simulink model "SCADA"  (R2021a)
settings: Solver=ode1  StartTime=0.0  StopTime=inf  FixedStep=0.001  RelTol=1e-3
InitFcn:
  | addpath('SCADA');
  | initFcn_SCADA;
model workspace (MAT data in the model file):
  RadSysCoeff = Simulink.Parameter
  RadSysCoeff.Value = [1 2 3 4]
  RadSysCoeff.DataType = 'auto'
  RadSysCoeff.Dimensions = [1 4]
values from neighbouring files (symbols this model uses):
  s = scatter(X(iVar),Y(iVar),100,[color(N-i+1,:)])    [postprocess_datafiles_accum_wRV.m]
undefined symbols (not defined in the file or in its folder): daq, g, HIL_act_A_cap, HIL_act_A_rod, HIL_charge_kd, HIL_charge_ki, HIL_charge_kp, HIL_charge_nMax, HIL_charge_nMin, HIL_ERU_kd, HIL_ERU_ki, HIL_ERU_kp, HIL_ERU_nMax, HIL_ERU_nMin, HIL_gen_kd, HIL_gen_ki, HIL_gen_kp, HIL_gen_nMax, HIL_gen_nMin, HIL_H1T_kp, HIL_H1T_negCutIn, HIL_H1T_posCutIn, HIL_scale_sys, HIL_WECpump_A_cap, HIL_WECpump_A_rod, HIL_WECpump_ang2lin, HIL_WECpump_negativeLimit, HIL_WECpump_positiveLimit, National_Instruments, PCIe, rho, wave_phi, wave_S_w, WEC_A_rad, WEC_B_rad, WEC_dw, WEC_F_amp, WEC_h, WEC_I, WEC_I_inf, WEC_ICs, WEC_L_cm, WEC_L_flap, WEC_m, WEC_phi_e, WEC_T, WEC_W, WEC_w
libraries: sldrtlib x21, daqlib x2, slpidlib x2, pid_lib x1, simulink x1
settings Model: Creator=Jeremy  LastModifiedBy=simmo536
settings RTWCC: BuildConfiguration=Faster Runs

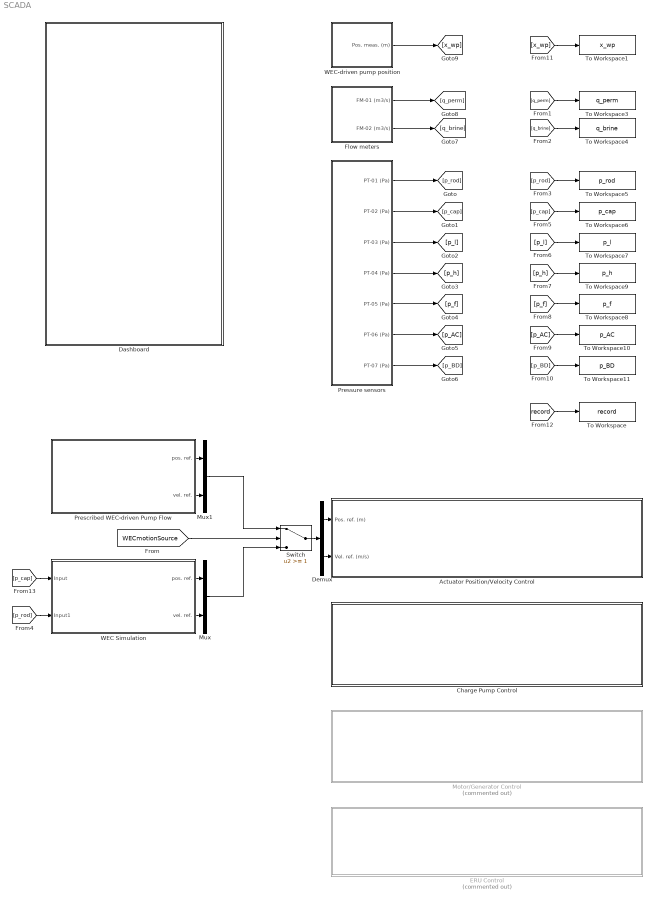
== system SCADA ==
  Actuator Position/Velocity Control : Subsystem
  Charge Pump Control : Subsystem
  Dashboard : Subsystem
  Demux : Demux  Outputs=2
  ERU Control : Subsystem  Commented=on
  Flow meters : Subsystem
  Motor/Generator Control : Subsystem  Commented=on
  Mux : Mux  Inputs=2
  Mux1 : Mux  Inputs=2
  Prescribed WEC-driven Pump Flow : Subsystem
  Pressure sensors : Subsystem
  Switch : Switch  Threshold=1
  To Workspace : ToWorkspace  VariableName=record  SaveFormat=Timeseries  SampleTime=-1
  To Workspace1 : ToWorkspace  VariableName=x_wp  SaveFormat=Timeseries  SampleTime=-1
  To Workspace10 : ToWorkspace  VariableName=p_AC  SaveFormat=Timeseries  SampleTime=-1
  To Workspace11 : ToWorkspace  VariableName=p_BD  SaveFormat=Timeseries  SampleTime=-1
  To Workspace3 : ToWorkspace  VariableName=q_perm  SaveFormat=Timeseries  SampleTime=-1
  To Workspace4 : ToWorkspace  VariableName=q_brine  SaveFormat=Timeseries  SampleTime=-1
  To Workspace5 : ToWorkspace  VariableName=p_rod  SaveFormat=Timeseries  SampleTime=-1
  To Workspace6 : ToWorkspace  VariableName=p_cap  SaveFormat=Timeseries  SampleTime=-1
  To Workspace7 : ToWorkspace  VariableName=p_l  SaveFormat=Timeseries  SampleTime=-1
  To Workspace8 : ToWorkspace  VariableName=p_f  SaveFormat=Timeseries  SampleTime=-1
  To Workspace9 : ToWorkspace  VariableName=p_h  SaveFormat=Timeseries  SampleTime=-1
  WEC Simulation : Subsystem
  WEC-driven pump position : Subsystem
  wires:
  WEC-driven pump position/1(Pos. meas. (m)) -> [x_wp]
  Pressure sensors/1(PT-01 (Pa)) -> [p_rod]
  Pressure sensors/2(PT-02 (Pa)) -> [p_cap]
  Pressure sensors/3(PT-03 (Pa)) -> [p_l]
  Pressure sensors/4(PT-04 (Pa)) -> [p_h]
  Pressure sensors/7(PT-07 (Pa)) -> [p_BD]
  Pressure sensors/6(PT-06 (Pa)) -> [p_AC]
  Pressure sensors/5(PT-05 (Pa)) -> [p_f]
  Flow meters/2(FM-02 (m3/s)) -> [q_brine]
  Flow meters/1(FM-01 (m3/s)) -> [q_perm]
  [record] -> To Workspace/1
  [x_wp] -> To Workspace1/1
  [q_perm] -> To Workspace3/1
  [p_rod] -> To Workspace5/1
  [q_brine] -> To Workspace4/1
  [p_cap] -> To Workspace6/1
  [p_l] -> To Workspace7/1
  [p_h] -> To Workspace9/1
  [p_f] -> To Workspace8/1
  [p_AC] -> To Workspace10/1
  [p_BD] -> To Workspace11/1
  [p_cap] -> WEC Simulation/1(Input)
  [p_rod] -> WEC Simulation/2(Input1)
  WEC Simulation/2(vel. ref.) -> Mux/2
  WEC Simulation/1(pos. ref.) -> Mux/1
  Demux/1 -> Actuator Position/Velocity Control/1(Pos. ref. (m))
  Demux/2 -> Actuator Position/Velocity Control/2(Vel. ref. (m/s))
  Switch/1 -> Demux/1
  [WECmotionSource] -> Switch/2
  Mux/1 -> Switch/3
  Prescribed WEC-driven Pump Flow/1(pos. ref.) -> Mux1/1
  Prescribed WEC-driven Pump Flow/2(vel. ref.) -> Mux1/2
  Mux1/1 -> Switch/1

== system SCADA/Actuator Position//Velocity Control ==
  Pos. ref. (m) : Inport
  Vel. ref. (m/s) : Inport  Port=2
  Derivative : Derivative
  Subsystem : Subsystem
  Transfer Fcn : TransferFcn  Denominator=[1/0.01 1]
  wires:
  [x_wp] -> Subsystem/3(Pos. meas. (m)), Derivative/1
  Derivative/1 -> Transfer Fcn/1
  Pos. ref. (m)/1 -> Subsystem/1(Pos. ref. (m))
  Vel. ref. (m/s)/1 -> Subsystem/2(Vel. ref. (m/s))
  Transfer Fcn/1 -> Subsystem/4(Vel. meas. (m/s))
  [H1T_shaftSpeed] -> Subsystem/5(H1T shaft speed (rpm))

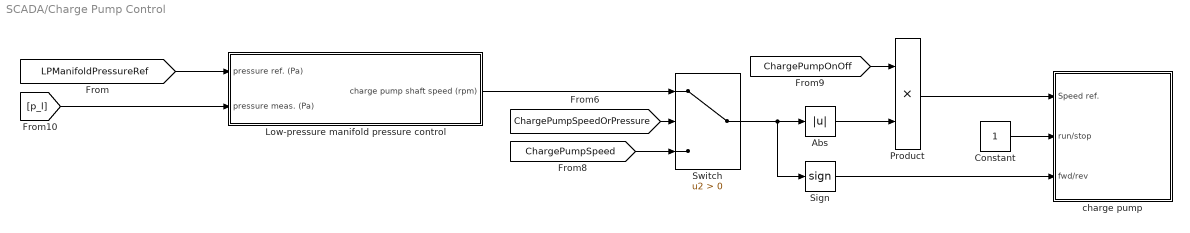
== system SCADA/Charge Pump Control ==
  Abs : Abs
  Constant : Constant
  Low-pressure manifold pressure control : Subsystem
  Product : Product
  Sign : Signum
  Switch : Switch  Criteria=u2 > Threshold
  charge pump : Subsystem
  wires:
  [p_l] -> Low-pressure manifold pressure control/2(pressure meas. (Pa))
  [ChargePumpSpeed] -> Switch/3
  Abs/1 -> Product/2
  Switch/1 -> Sign/1, Abs/1
  [LPManifoldPressureRef] -> Low-pressure manifold pressure control/1(pressure ref. (Pa))
  [ChargePumpOnOff] -> Product/1
  Low-pressure manifold pressure control/1(charge pump shaft speed (rpm)) -> Switch/1
  [ChargePumpSpeedOrPressure] -> Switch/2
  Product/1 -> charge pump/1(Speed ref.)
  Sign/1 -> charge pump/3(fwd/rev)
  Constant/1 -> charge pump/2(run/stop)

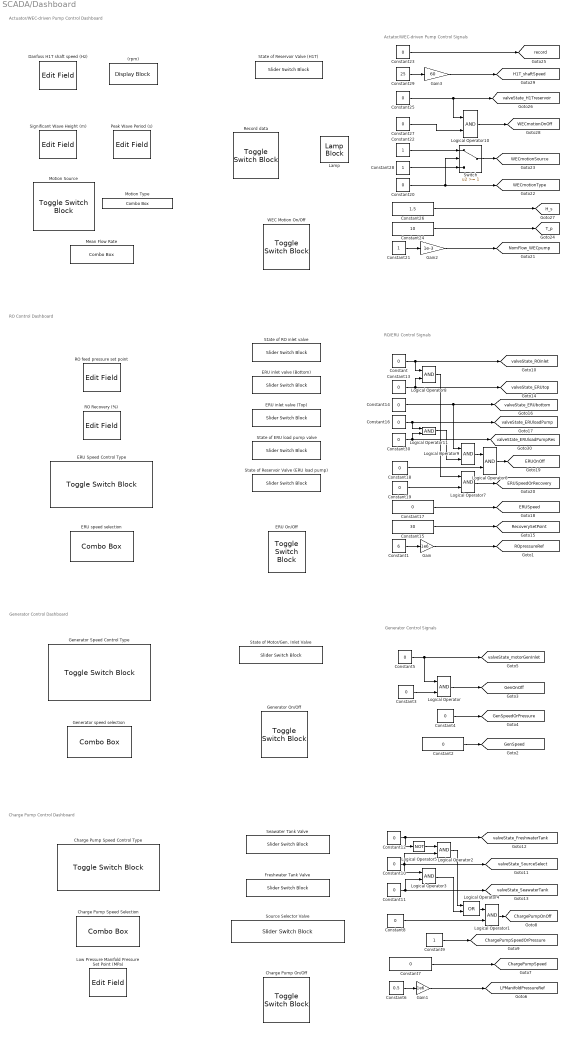
== system SCADA/Dashboard ==
  note: Charge Pump Control Dashboard
  note: Generator Control Signals
  note: RO Control Dashboard
  note: Generator Control Dashboard
  note: RO/ERU Control Signals
  note: Actuator/WEC-driven Pump Control Dashboard
  note: Actator/WEC-driven Pump Control Signals
  (rpm) : DisplayBlock  LabelPosition=Hide  Transparency=1
  Charge Pump On/Off : ToggleSwitchBlock  LabelPosition=Hide
      settings: Values={{'Off', 'On'}, [0 1]}
  Charge Pump Speed Control Type : ToggleSwitchBlock  LabelPosition=Hide
      settings: Values={{'Pressure control', 'Speed control'}, [1 0]}
  Charge Pump Speed Selection : ComboBox  LabelPosition=Hide  SelectedLabel=0 rpm
      settings: Values={{'0 rpm', '700 rpm', '1250 rpm', '2000 rpm', '2650 rpm', '3300 rpm'}, [0 700 1350 2000 2650 3300]}
  Constant{,2..5,7..8,10..14,16..20,23,25,27,30} (21 alike) : Constant  Value=0
  Constant1 : Constant  Value=6
  Constant15 : Constant  Value=30
  Constant{9,21..22,28} (4 alike) : Constant
  Constant24 : Constant  Value=10
  Constant26 : Constant  Value=1.5
  Constant29 : Constant  Value=25
  Constant6 : Constant  Value=0.5
  Danfoss H1T shaft speed (Hz) : EditField  LabelPosition=Hide  ShowInitialText=on  Alignment=Center
  ERU On/Off : ToggleSwitchBlock  LabelPosition=Hide
      settings: Values={{'Off', 'On'}, [0 1]}
  ERU Speed Control Type : ToggleSwitchBlock  LabelPosition=Hide
      settings: Values={{'Recovery control', 'Speed control'}, [1 0]}
  ERU inlet valve (Bottom) : SliderSwitchBlock  LabelPosition=Hide
      settings: Values={{'Closed', 'Open'}, [0 1]}
  ERU inlet valve (Top) : SliderSwitchBlock  LabelPosition=Hide
      settings: Values={{'Closed', 'Open'}, [0 1]}
  ERU speed selection : ComboBox  LabelPosition=Hide  SelectedLabel=0 rpm
      settings: Values={{'0 rpm', '500 rpm', '1000 rpm'}, [0 500 1000]}
  Freshwater Tank Valve : SliderSwitchBlock  LabelPosition=Hide
      settings: Values={{'Closed', 'Open'}, [0 1]}
  Gain : Gain  Gain=1e6
  Gain1 : Gain  Gain=1e6
  Gain2 : Gain  Gain=1e-3
  Gain3 : Gain  Gain=60
  Generator On/Off : ToggleSwitchBlock  LabelPosition=Hide
      settings: Values={{'Off', 'On'}, [0 1]}
  Generator Speed Control Type : ToggleSwitchBlock  LabelPosition=Hide
      settings: Values={{'Pressure control', 'Speed control'}, [1 0]}
  Generator speed selection : ComboBox  LabelPosition=Hide  SelectedLabel=0 rpm
      settings: Values={{'0 rpm', '500 rpm', '1000 rpm'}, [0 500 1000]}
  Lamp : LampBlock  LabelPosition=Hide
  Logical Operator{,1..3,6..11} (10 alike) : Logic  AllPortsSameDT=off  OutDataTypeStr=boolean
  Logical Operator4 : Logic  Operator=OR  AllPortsSameDT=off  OutDataTypeStr=boolean
  Logical Operator5 : Logic  Operator=NOT  AllPortsSameDT=off  OutDataTypeStr=boolean
  Low Pressure Manifold Pressure Set Point (MPa) : EditField  LabelPosition=Hide  ShowInitialText=on  Alignment=Center
  Mean Flow Rate : ComboBox  LabelPosition=Hide  SelectedLabel=1 L/s
      settings: Values={{'0 L/s', '1 L/s', '2 L/2'}, [0 1 2]}
  Motion Source : ToggleSwitchBlock  LabelPosition=Hide
      settings: Values={{'Prescribed', 'Simulation'}, [1 0]}
  Motion Type : ComboBox  LabelPosition=Hide  SelectedLabel=Constant Velocity
      settings: Values={{'Constant Velocity', 'Regular Waves', 'Irregular Waves'}, [0 1 2]}
  Peak Wave Period (s) : EditField  LabelPosition=Hide  ShowInitialText=on  Alignment=Center
  RO Recovery (%) : EditField  LabelPosition=Hide  ShowInitialText=on  Alignment=Center
  RO feed pressure set point : EditField  LabelPosition=Hide  ShowInitialText=on  Alignment=Center
  Record data : ToggleSwitchBlock  LabelPosition=Hide
      settings: Values={{'Off', 'On'}, [0 1]}
  Seawater Tank Valve : SliderSwitchBlock  LabelPosition=Hide
      settings: Values={{'Closed', 'Open'}, [0 1]}
  Significant Wave Height (m) : EditField  LabelPosition=Hide  ShowInitialText=on  Alignment=Center
  Source Selector Valve : SliderSwitchBlock  LabelPosition=Hide
      settings: Values={{'Freshwater', 'Seawater'}, [0 1]}
  State of ERU load pump valve : SliderSwitchBlock  LabelPosition=Hide
      settings: Values={{'Closed', 'Open'}, [0 1]}
  State of Motor/Gen. Inlet Valve : SliderSwitchBlock  LabelPosition=Hide
      settings: Values={{'Closed', 'Open'}, [0 1]}
  State of RO inlet valve : SliderSwitchBlock  LabelPosition=Hide
      settings: Values={{'Closed', 'Open'}, [0 1]}
  State of Reservoir Valve (ERU load pump) : SliderSwitchBlock  LabelPosition=Hide
      settings: Values={{'Closed', 'Open'}, [0 1]}
  State of Reservoir Valve (H1T) : SliderSwitchBlock  LabelPosition=Hide
      settings: Values={{'Closed', 'Open'}, [0 1]}
  Switch : Switch  Threshold=1
  WEC Motion On/Off : ToggleSwitchBlock  LabelPosition=Hide
      settings: Values={{'Off', 'On'}, [0 1]}
  tag scope: ChargePumpOnOff=global, ChargePumpSpeed=global, ChargePumpSpeedOrPressure=global, ERUOnOff=global, ERUSpeed=global, ERUSpeedOrRecovery=global, GenOnOff=global, GenSpeed=global, GenSpeedOrPressure=global, H1T_shaftSpeed=global, H_s=global, LPManifoldPressureRef=global, NomFlow_WECpump=global, ROpressureRef=global, RecoverySetPoint=global, T_p=global, WECmotionOnOff=global, WECmotionSource=global, WECmotionType=global, record=global, valveState_ERUbottom=global, valveState_ERUloadPump=global, valveState_ERUloadPumpRes=global, valveState_ERUtop=global, valveState_FreshwaterTank=global, valveState_H1Treservoir=global, valveState_ROinlet=global, valveState_SeawaterTank=global, valveState_SourceSelect=global, valveState_motorGenInlet=global
  wires:
  Constant/1 -> Logical Operator8/1, [valveState_ROinlet]
  Constant1/1 -> Gain/1
  Gain/1 -> [ROpressureRef]
  Constant2/1 -> [GenSpeed]
  Constant3/1 -> Logical Operator/2
  Constant4/1 -> [GenSpeedOrPressure]
  Constant5/1 -> Logical Operator/1, [valveState_motorGenInlet]
  Logical Operator/1 -> [GenOnOff]
  Logical Operator1/1 -> [ChargePumpOnOff]
  Constant9/1 -> [ChargePumpSpeedOrPressure]
  Constant10/1 -> [valveState_SourceSelect], Logical Operator2/2, Logical Operator3/1
  Gain1/1 -> [LPManifoldPressureRef]
  Constant6/1 -> Gain1/1
  Constant8/1 -> Logical Operator1/2
  Constant7/1 -> [ChargePumpSpeed]
  Constant12/1 -> Logical Operator5/1, [valveState_FreshwaterTank]
  Constant11/1 -> Logical Operator3/2, [valveState_SeawaterTank]
  Logical Operator4/1 -> Logical Operator1/1
  Logical Operator3/1 -> Logical Operator4/2
  Logical Operator2/1 -> Logical Operator4/1
  Logical Operator5/1 -> Logical Operator2/1
  Logical Operator6/1 -> [ERUOnOff]
  Constant17/1 -> [ERUSpeed]
  Constant13/1 -> Logical Operator8/2, [valveState_ERUtop]
  Constant19/1 -> Logical Operator7/2
  Constant18/1 -> Logical Operator6/2
  Constant14/1 -> [valveState_ERUbottom], Logical Operator9/1
  Constant15/1 -> [RecoverySetPoint]
  Logical Operator7/1 -> [ERUSpeedOrRecovery]
  Logical Operator8/1 -> Logical Operator7/1
  Logical Operator9/1 -> Logical Operator6/1
  Constant16/1 -> [valveState_ERUloadPump], Logical Operator11/1
  Constant24/1 -> [T_p]
  Constant26/1 -> [H_s]
  Logical Operator10/1 -> [WECmotionOnOff]
  Constant21/1 -> Gain2/1
  Constant25/1 -> Logical Operator10/1, [valveState_H1Treservoir]
  Gain2/1 -> [NomFlow_WECpump]
  Constant27/1 -> Logical Operator10/2
  Constant20/1 -> Switch/2, [WECmotionType]
  Constant22/1 -> Switch/1
  Constant23/1 -> [record]
  Constant28/1 -> Switch/3
  Switch/1 -> [WECmotionSource]
  Constant29/1 -> Gain3/1
  Gain3/1 -> [H1T_shaftSpeed]
  Constant30/1 -> [valveState_ERUloadPumpRes], Logical Operator11/2
  Logical Operator11/1 -> Logical Operator9/2

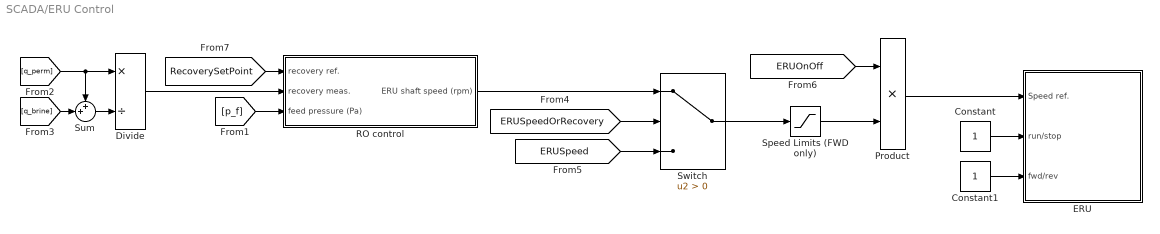
== system SCADA/ERU Control ==
  Constant : Constant
  Constant1 : Constant
  Divide : Product  Inputs=*/
  ERU : Subsystem
  Product : Product
  RO control : Subsystem
  Speed Limits (FWD only) : Saturate  UpperLimit=HIL_ERU_nMax  LowerLimit=HIL_ERU_nMin
  Sum : Sum  Inputs=++|
  Switch : Switch  Criteria=u2 > Threshold
  wires:
  Constant/1 -> ERU/2(run/stop)
  [p_f] -> RO control/3(feed pressure (Pa))
  [q_perm] -> Sum/1, Divide/1
  [q_brine] -> Sum/2
  Sum/1 -> Divide/2
  [RecoverySetPoint] -> RO control/1(recovery ref.)
  Divide/1 -> RO control/2(recovery meas.)
  [ERUSpeedOrRecovery] -> Switch/2
  Switch/1 -> Speed Limits (FWD only)/1
  [ERUSpeed] -> Switch/3
  RO control/1(ERU shaft speed (rpm)) -> Switch/1
  Speed Limits (FWD only)/1 -> Product/2
  [ERUOnOff] -> Product/1
  Product/1 -> ERU/1(Speed ref.)
  Constant1/1 -> ERU/3(fwd/rev)

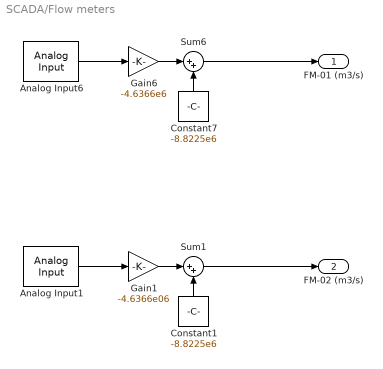
== system SCADA/Flow meters ==
  Analog Input1 : sldrtlib/Analog Input  SampleTime=0.1  MaxMissedTicks=10  ShowMissedTicks=off  YieldWhenWaiting=on  DrvName=National_Instruments/PCIe-6343  DrvAddress=4294967295  DrvOptions=[0 4367 12288 3 3 3 3]  Channels=7  RangeMode=1  VoltRange=1  DataType=1
      settings: AttributesFormatString=National Instruments\nPCIe-6343 [auto]
  Analog Input6 : sldrtlib/Analog Input  SampleTime=0.1  MaxMissedTicks=10  ShowMissedTicks=off  YieldWhenWaiting=on  DrvName=National_Instruments/PCIe-6343  DrvAddress=4294967295  DrvOptions=[0 4367 12288 3 3 3 3]  Channels=7  RangeMode=1  VoltRange=1  DataType=1
      settings: AttributesFormatString=National Instruments\nPCIe-6343 [auto]
  Constant1 : Constant  Value=-8.8225e6
  Constant7 : Constant  Value=-8.8225e6
  Gain1 : Gain  Gain=-4.6366e06
  Gain6 : Gain  Gain=-4.6366e6
  Sum1 : Sum  Inputs=|++
  Sum6 : Sum  Inputs=|++
  FM-01 (m3/s) : Outport
  FM-02 (m3/s) : Outport  Port=2
  wires:
  Constant7/1 -> Sum6/2
  Analog Input6/1 -> Gain6/1
  Gain6/1 -> Sum6/1
  Sum6/1 -> FM-01 (m3/s)/1
  Gain1/1 -> Sum1/1
  Sum1/1 -> FM-02 (m3/s)/1
  Constant1/1 -> Sum1/2
  Analog Input1/1 -> Gain1/1

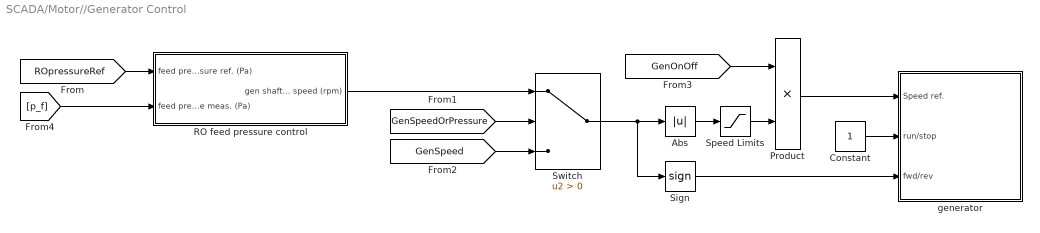
== system SCADA/Motor//Generator Control ==
  Abs : Abs
  Constant : Constant
  Product : Product
  RO feed pressure control : Subsystem
  Sign : Signum
  Speed Limits : Saturate  UpperLimit=HIL_gen_nMax  LowerLimit=HIL_gen_nMin
  Switch : Switch  Criteria=u2 > Threshold
  generator : Subsystem
  wires:
  RO feed pressure control/1(gen shaft speed (rpm)) -> Switch/1
  [p_f] -> RO feed pressure control/2(feed pressure meas. (Pa))
  [ROpressureRef] -> RO feed pressure control/1(feed pressure ref. (Pa))
  Switch/1 -> Sign/1, Abs/1
  [GenSpeedOrPressure] -> Switch/2
  [GenSpeed] -> Switch/3
  [GenOnOff] -> Product/1
  Product/1 -> generator/1(Speed ref.)
  Constant/1 -> generator/2(run/stop)
  Sign/1 -> generator/3(fwd/rev)
  Speed Limits/1 -> Product/2
  Abs/1 -> Speed Limits/1

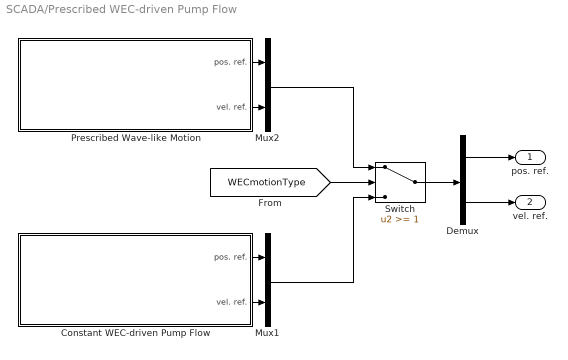
== system SCADA/Prescribed WEC-driven Pump Flow ==
  Constant WEC-driven Pump Flow : Subsystem
  Demux : Demux  Outputs=2
  Mux1 : Mux  Inputs=2
  Mux2 : Mux  Inputs=2
  Prescribed Wave-like Motion : Subsystem
  Switch : Switch  Threshold=1
  pos. ref. : Outport
  vel. ref. : Outport  Port=2
  wires:
  Prescribed Wave-like Motion/2(vel. ref.) -> Mux2/2
  Prescribed Wave-like Motion/1(pos. ref.) -> Mux2/1
  Mux2/1 -> Switch/1
  Demux/2 -> vel. ref./1
  Demux/1 -> pos. ref./1
  Constant WEC-driven Pump Flow/1(pos. ref.) -> Mux1/1
  Constant WEC-driven Pump Flow/2(vel. ref.) -> Mux1/2
  [WECmotionType] -> Switch/2
  Switch/1 -> Demux/1
  Mux1/1 -> Switch/3

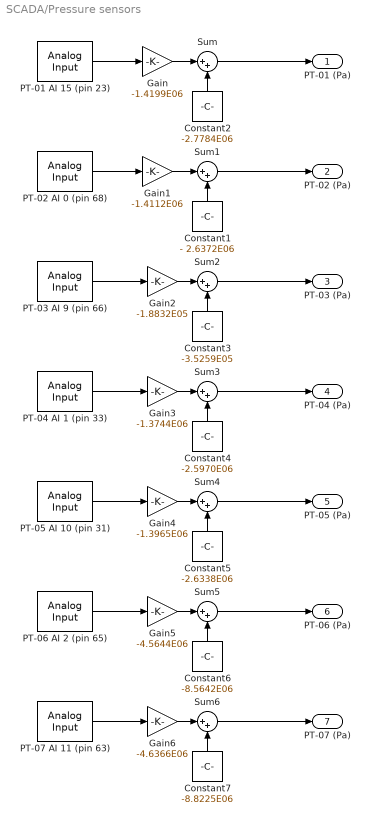
== system SCADA/Pressure sensors ==
  Constant1 : Constant  Value=- 2.6372E06
  Constant2 : Constant  Value=-2.7784E06
  Constant3 : Constant  Value=-3.5259E05
  Constant4 : Constant  Value=-2.5970E06
  Constant5 : Constant  Value=-2.6338E06
  Constant6 : Constant  Value=-8.5642E06
  Constant7 : Constant  Value=-8.8225E06
  Gain : Gain  Gain=-1.4199E06
  Gain1 : Gain  Gain=-1.4112E06
  Gain2 : Gain  Gain=-1.8832E05
  Gain3 : Gain  Gain=-1.3744E06
  Gain4 : Gain  Gain=-1.3965E06
  Gain5 : Gain  Gain=-4.5644E06
  Gain6 : Gain  Gain=-4.6366E06
  PT-01 AI 15 (pin 23) : sldrtlib/Analog Input  SampleTime=0.001  MaxMissedTicks=inf  ShowMissedTicks=off  YieldWhenWaiting=on  DrvName=National_Instruments/PCIe-6343  DrvAddress=4294967295  DrvOptions=[0 4367 12288 3 3 3 3]  Channels=16  RangeMode=1  VoltRange=1  DataType=1
      settings: AttributesFormatString=National Instruments\nPCIe-6343 [auto]
  PT-02 AI 0 (pin 68) : sldrtlib/Analog Input  SampleTime=0.1  MaxMissedTicks=inf  ShowMissedTicks=off  YieldWhenWaiting=on  DrvName=National_Instruments/PCIe-6343  DrvAddress=4294967295  DrvOptions=[0 4367 12288 3 3 3 3]  Channels=1  RangeMode=1  VoltRange=1  DataType=1
      settings: AttributesFormatString=National Instruments\nPCIe-6343 [auto]
  PT-03 AI 9 (pin 66) : sldrtlib/Analog Input  SampleTime=0.1  MaxMissedTicks=inf  ShowMissedTicks=off  YieldWhenWaiting=on  DrvName=National_Instruments/PCIe-6343  DrvAddress=4294967295  DrvOptions=[0 4367 12288 3 3 3 3]  Channels=10  RangeMode=1  VoltRange=1  DataType=1
      settings: AttributesFormatString=National Instruments\nPCIe-6343 [auto]
  PT-04 AI 1 (pin 33) : sldrtlib/Analog Input  SampleTime=0.1  MaxMissedTicks=10  ShowMissedTicks=off  YieldWhenWaiting=on  DrvName=National_Instruments/PCIe-6343  DrvAddress=4294967295  DrvOptions=[0 4367 12288 3 3 3 3]  Channels=2  RangeMode=1  VoltRange=1  DataType=1
      settings: AttributesFormatString=National Instruments\nPCIe-6343 [auto]
  PT-05 AI 10 (pin 31) : sldrtlib/Analog Input  SampleTime=0.1  MaxMissedTicks=inf  ShowMissedTicks=off  YieldWhenWaiting=on  DrvName=National_Instruments/PCIe-6343  DrvAddress=4294967295  DrvOptions=[0 4367 12288 3 3 3 3]  Channels=11  RangeMode=1  VoltRange=1  DataType=1
      settings: AttributesFormatString=National Instruments\nPCIe-6343 [auto]
  PT-06 AI 2 (pin 65) : sldrtlib/Analog Input  SampleTime=0.1  MaxMissedTicks=10  ShowMissedTicks=off  YieldWhenWaiting=on  DrvName=National_Instruments/PCIe-6343  DrvAddress=4294967295  DrvOptions=[0 4367 12288 3 3 3 3]  Channels=3  RangeMode=1  VoltRange=1  DataType=1
      settings: AttributesFormatString=National Instruments\nPCIe-6343 [auto]
  PT-07 AI 11 (pin 63) : sldrtlib/Analog Input  SampleTime=0.1  MaxMissedTicks=10  ShowMissedTicks=off  YieldWhenWaiting=on  DrvName=National_Instruments/PCIe-6343  DrvAddress=4294967295  DrvOptions=[0 4367 12288 3 3 3 3]  Channels=12  RangeMode=1  VoltRange=1  DataType=1
      settings: AttributesFormatString=National Instruments\nPCIe-6343 [auto]
  Sum{,1..6} (7 alike) : Sum  Inputs=|++
  PT-01 (Pa) : Outport
  PT-02 (Pa) : Outport  Port=2
  PT-03 (Pa) : Outport  Port=3
  PT-04 (Pa) : Outport  Port=4
  PT-05 (Pa) : Outport  Port=5
  PT-06 (Pa) : Outport  Port=6
  PT-07 (Pa) : Outport  Port=7
  wires:
  PT-01 AI 15 (pin 23)/1 -> Gain/1
  Constant2/1 -> Sum/2
  Sum/1 -> PT-01 (Pa)/1
  Sum1/1 -> PT-02 (Pa)/1
  Sum2/1 -> PT-03 (Pa)/1
  Sum3/1 -> PT-04 (Pa)/1
  Sum4/1 -> PT-05 (Pa)/1
  Sum5/1 -> PT-06 (Pa)/1
  Gain/1 -> Sum/1
  PT-02 AI 0 (pin 68)/1 -> Gain1/1
  Constant1/1 -> Sum1/2
  Gain1/1 -> Sum1/1
  PT-03 AI 9 (pin 66)/1 -> Gain2/1
  Constant3/1 -> Sum2/2
  Gain2/1 -> Sum2/1
  PT-04 AI 1 (pin 33)/1 -> Gain3/1
  Constant4/1 -> Sum3/2
  Gain3/1 -> Sum3/1
  PT-05 AI 10 (pin 31)/1 -> Gain4/1
  Constant5/1 -> Sum4/2
  Gain4/1 -> Sum4/1
  PT-06 AI 2 (pin 65)/1 -> Gain5/1
  Constant6/1 -> Sum5/2
  Gain5/1 -> Sum5/1
  PT-07 AI 11 (pin 63)/1 -> Gain6/1
  Sum6/1 -> PT-07 (Pa)/1
  Constant7/1 -> Sum6/2
  Gain6/1 -> Sum6/1

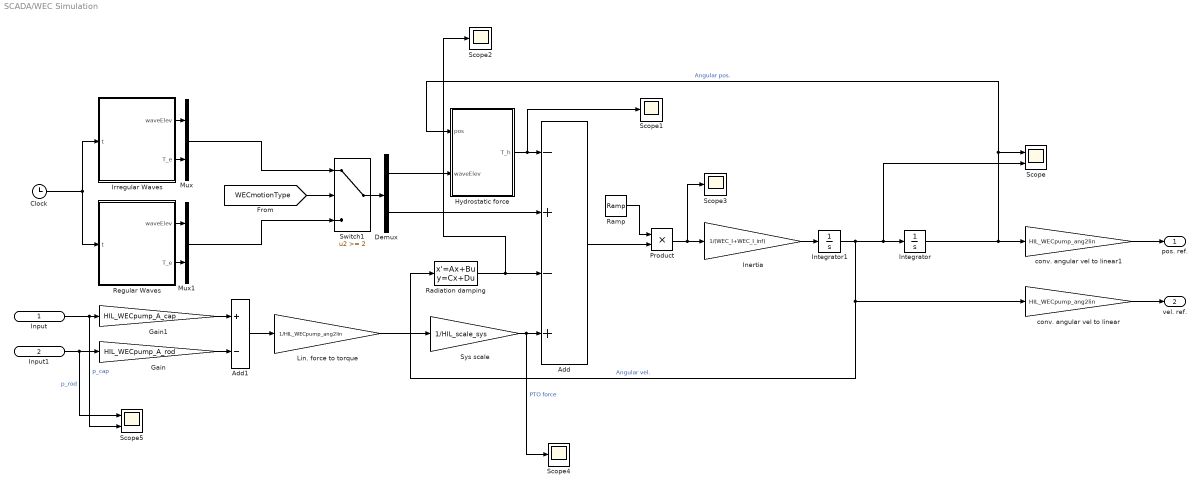
== system SCADA/WEC Simulation ==
  Input : Inport
  Input1 : Inport  Port=2
  Add : Sum  Inputs=-+-+
  Add1 : Sum  Inputs=+-
  Clock : Clock
  Demux : Demux  Outputs=2
  Gain : Gain  Gain=HIL_WECpump_A_rod
  Gain1 : Gain  Gain=HIL_WECpump_A_cap
  Hydrostatic force : MATLAB Function  TreatAsAtomicUnit=on
  Inertia : Gain  Gain=1/(WEC_I+WEC_I_inf)
  Integrator : Integrator
  Integrator1 : Integrator
  Irregular Waves : MATLAB Function  TreatAsAtomicUnit=on
  Lin. force to torque : Gain  Gain=1/HIL_WECpump_ang2lin
  Mux : Mux  Inputs=2
  Mux1 : Mux  Inputs=2
  Product : Product
  Radiation damping : StateSpace  A=WEC_A_rad  B=WEC_B_rad  C=[1,0,0]  D=0  InitialCondition=WEC_ICs
  Ramp : simulink/Sources/Ramp  slope=1/5  start=5  InitialOutput=0
  Regular Waves : MATLAB Function  TreatAsAtomicUnit=on
  Scope : Scope  NumInputPorts=2
  Scope{1..4} (4 alike) : Scope
  Scope5 : Scope  NumInputPorts=2
  Switch1 : Switch  Threshold=2
  Sys scale : Gain  Gain=1/HIL_scale_sys
  conv. angular vel to linear : Gain  Gain=HIL_WECpump_ang2lin
  conv. angular vel to linear1 : Gain  Gain=HIL_WECpump_ang2lin
  pos. ref. : Outport
  vel. ref. : Outport  Port=2
  wires:
  Radiation damping/1 -> Scope2/1, Add/3
  Clock/1 -> Regular Waves/1(t), Irregular Waves/1(t)
  Irregular Waves/1(waveElev) -> Mux/1
  Irregular Waves/2(T_e) -> Mux/2
  Hydrostatic force/1(T_h) -> Scope1/1, Add/1
  Inertia/1 -> Integrator1/1
  Integrator1/1 -> Scope/2, Integrator/1, Radiation damping/1, conv. angular vel to linear/1  "Angular vel."
  Integrator/1 -> conv. angular vel to linear1/1, Scope/1, Hydrostatic force/1(pos)  "Angular pos."
  Lin. force to torque/1 -> Sys scale/1
  Add1/1 -> Lin. force to torque/1
  Input/1 -> Scope5/2, Gain1/1  "p_cap"
  Input1/1 -> Scope5/1, Gain/1  "p_rod"
  conv. angular vel to linear1/1 -> pos. ref./1
  conv. angular vel to linear/1 -> vel. ref./1
  Sys scale/1 -> Scope4/1, Add/4  "PTO force"
  Gain/1 -> Add1/2
  Gain1/1 -> Add1/1
  Demux/1 -> Hydrostatic force/2(waveElev)
  [WECmotionType] -> Switch1/2
  Demux/2 -> Add/2
  Regular Waves/1(waveElev) -> Mux1/1
  Regular Waves/2(T_e) -> Mux1/2
  Switch1/1 -> Demux/1
  Mux1/1 -> Switch1/3
  Mux/1 -> Switch1/1
  Product/1 -> Scope3/1, Inertia/1
  Add/1 -> Product/2
  Ramp/1 -> Product/1

== system SCADA/WEC-driven pump position ==
  Analog Input : sldrtlib/Analog Input  SampleTime=0.1  MaxMissedTicks=inf  ShowMissedTicks=off  YieldWhenWaiting=on  DrvName=National_Instruments/PCIe-6343  DrvAddress=4294967295  DrvOptions=[0 4367 12288 3 3 3 3]  Channels=7  RangeMode=1  VoltRange=1  DataType=1
      settings: AttributesFormatString=National Instruments\nPCIe-6343 [auto]
  Constant2 : Constant  Value=2.5
  Gain : Gain  Gain=.1013
  Scope : Scope
  Sum : Sum  Inputs=|+-
  Pos. meas. (m) : Outport
  wires:
  Constant2/1 -> Sum/2
  Sum/1 -> Gain/1
  Gain/1 -> Pos. meas. (m)/1  "Pos (m)"
  Analog Input/1 -> Scope/1, Sum/1

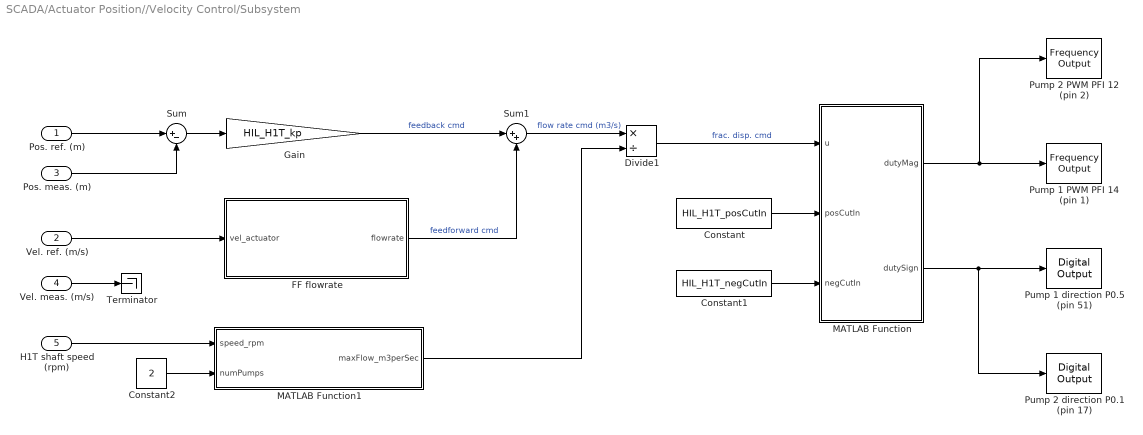
== system SCADA/Actuator Position//Velocity Control/Subsystem ==
  Pos. ref. (m) : Inport
  Vel. ref. (m/s) : Inport  Port=2
  Pos. meas. (m) : Inport  Port=3
  Vel. meas. (m/s) : Inport  Port=4
  H1T shaft speed (rpm) : Inport  Port=5
  Constant : Constant  Value=HIL_H1T_posCutIn
  Constant1 : Constant  Value=HIL_H1T_negCutIn
  Constant2 : Constant  Value=2
  Divide1 : Product  Inputs=*/
  FF flowrate : MATLAB Function  TreatAsAtomicUnit=on
  Gain : Gain  Gain=HIL_H1T_kp
  MATLAB Function : MATLAB Function  TreatAsAtomicUnit=on
  MATLAB Function1 : MATLAB Function  TreatAsAtomicUnit=on
  Pump 1 PWM PFI 14 (pin 1) : sldrtlib/Frequency Output  SampleTime=0.1  MaxMissedTicks=inf  ShowMissedTicks=off  YieldWhenWaiting=off  DrvName=National_Instruments/PCIe-6343  DrvAddress=4294967295  DrvOptions=[0 4367 12288 3 3 3 3]  Channels=3  FrequencySource=1  Frequency=100  FrequencyFinalValue=[]  DutySource=2  Duty=0  DutyFinalValue=0
      settings: AttributesFormatString=National Instruments\nPCIe-6343 [auto]  SourceProductBaseCode=WT
  Pump 1 direction P0.5 (pin 51) : sldrtlib/Digital Output  SampleTime=0.1  MaxMissedTicks=10  ShowMissedTicks=off  YieldWhenWaiting=off  DrvName=National_Instruments/PCIe-6343  DrvAddress=4294967295  DrvOptions=[0 4367 12288 3 3 3 3]  Channels=6  BitMode=1  InitialValue=1  FinalValue=1
      settings: AttributesFormatString=National Instruments\nPCIe-6343 [auto]  SourceProductBaseCode=WT
  Pump 2 PWM PFI 12 (pin 2) : sldrtlib/Frequency Output  SampleTime=0.1  MaxMissedTicks=inf  ShowMissedTicks=off  YieldWhenWaiting=off  DrvName=National_Instruments/PCIe-6343  DrvAddress=4294967295  DrvOptions=[0 4367 12288 3 3 3 3]  Channels=2  FrequencySource=1  Frequency=100  FrequencyFinalValue=[]  DutySource=2  Duty=0  DutyFinalValue=0
      settings: AttributesFormatString=National Instruments\nPCIe-6343 [auto]  SourceProductBaseCode=WT
  Pump 2 direction P0.1 (pin 17) : sldrtlib/Digital Output  SampleTime=0.1  MaxMissedTicks=10  ShowMissedTicks=off  YieldWhenWaiting=off  DrvName=National_Instruments/PCIe-6343  DrvAddress=4294967295  DrvOptions=[0 4367 12288 3 3 3 3]  Channels=1  BitMode=1  InitialValue=0  FinalValue=0
      settings: AttributesFormatString=National Instruments\nPCIe-6343 [auto]  SourceProductBaseCode=WT
  Sum : Sum  Inputs=|+-
  Sum1 : Sum  Inputs=|++
  Terminator : Terminator
  wires:
  FF flowrate/1(flowrate) -> Sum1/2  "feedforward cmd"
  Pos. meas. (m)/1 -> Sum/2
  MATLAB Function1/1(maxFlow_m3perSec) -> Divide1/2
  Constant2/1 -> MATLAB Function1/2(numPumps)
  Divide1/1 -> MATLAB Function/1(u)  "frac. disp. cmd"
  H1T shaft speed (rpm)/1 -> MATLAB Function1/1(speed_rpm)
  MATLAB Function/1(dutyMag) -> Pump 1 PWM PFI 14 (pin 1)/1, Pump 2 PWM PFI 12 (pin 2)/1
  Constant1/1 -> MATLAB Function/3(negCutIn)
  Sum1/1 -> Divide1/1  "flow rate cmd (m3/s)"
  Pos. ref. (m)/1 -> Sum/1
  Vel. ref. (m/s)/1 -> FF flowrate/1(vel_actuator)
  Gain/1 -> Sum1/1  "feedback cmd"
  MATLAB Function/2(dutySign) -> Pump 2 direction P0.1 (pin 17)/1, Pump 1 direction P0.5 (pin 51)/1
  Vel. meas. (m/s)/1 -> Terminator/1
  Sum/1 -> Gain/1
  Constant/1 -> MATLAB Function/2(posCutIn)

== system SCADA/Charge Pump Control/Low-pressure manifold pressure control ==
  pressure ref. (Pa) : Inport
  pressure meas. (Pa) : Inport  Port=2
  PID Controller : pid_lib/PID Controller  Controller=PI  Form=Parallel  TimeDomain=Continuous-time  UseExternalTs=off  SampleTime=-1  IntegratorMethod=Forward Euler  FilterMethod=Forward Euler  ControllerParametersSource=internal  P=HIL_charge_kp  I=HIL_charge_ki  D=HIL_charge_kd  UseFilter=on  N=100  TunerSelectOption=Transfer Function Based (PID Tuner App)  InitialConditionSource=internal  InitialConditionForIntegrator=0  InitialConditionForFilter=0  DifferentiatorICPrevScaledInput=0  ExternalReset=none  TrackingMode=off  Kt=1  LimitOutput=off  SatLimitsSource=internal  UpperSaturationLimit=inf  LowerSaturationLimit=-inf  LinearizeAsGain=on  AntiWindupMode=none  Kb=1  POutMin=[]  POutMax=[]  IOutMin=[]  IOutMax=[]  DOutMin=[]  DOutMax=[]  NOutMin=[]  NOutMax=[]  SumOutMin=[]  SumOutMax=[]  SaturationOutMin=[]  SaturationOutMax=[]  PParamMin=[]  PParamMax=[]  IParamMin=[]  IParamMax=[]  DParamMin=[]  DParamMax=[]  NParamMin=[]  NParamMax=[]  KbParamMin=[]  KbParamMax=[]  KtParamMin=[]  KtParamMax=[]  KbOutMin=[]  KbOutMax=[]  KtOutMin=[]  KtOutMax=[]  IntegratorOutMin=[]  IntegratorOutMax=[]  FilterOutMin=[]  FilterOutMax=[]  SumI1OutMin=[]  SumI1OutMax=[]  SumI2OutMin=[]  SumI2OutMax=[]  SumI3OutMin=[]  SumI3OutMax=[]  SumI4OutMin=[]  SumI4OutMax=[]  SumDOutMin=[]  SumDOutMax=[]  DifferentiatorOutMin=[]  DifferentiatorOutMax=[]  FilterDiffOutCoefMin=[]  FilterDiffOutCoefMax=[]  ReciprocalOutMin=[]  ReciprocalOutMax=[]  SumDenOutMin=[]  SumDenOutMax=[]  SumNumOutMin=[]  SumNumOutMax=[]  DivideOutMin=[]  DivideOutMax=[]  UdiffTsProdOutMin=[]  UdiffTsProdOutMax=[]  NTsProdOutMin=[]  NTsProdOutMax=[]  UintegralTsProdOutMin=[]  UintegralTsProdOutMax=[]  UngainTsProdOutMin=[]  UngainTsProdOutMax=[]  IntegratorContinuousStateAttributes=''  IntegratorStateMustResolveToSignalObject=off  IntegratorRTWStateStorageClass=Auto  FilterContinuousStateAttributes=''  FilterStateMustResolveToSignalObject=off  FilterRTWStateStorageClass=Auto  ParallelPVariant=InternalParameters  IdealPVariant=Disabled  IVariant=InternalParameters  DVariant=Disabled  IntegratorVariant=Continuous  SatVariant=Disabled  AWVariant=Passthrough  PCopyVariant=Disabled  TRVariant=Disabled  FdbkBlocksVariant=Forward  IdealPFdbkVariant=Disabled  SatFdbkVariant=Disabled  DerivativeFilterVariant=Disabled  NVariant=Disabled  NCopyVariant=Disabled_SignalSpec  FilterICVariant=Disabled  IntegratorICVariant=InternalICs  ExternalResetVariant=Disabled  TRSumVariant=Passthrough  SumFdbkVariant=Disabled  SumVariant=Sum_PI  TsampFilterVariant=InternalTs  TsampNgainVariant=Passthrough  TsampIntegralVariant=Passthrough  ExternalSaturationOutDataTypeStr=Inherit: Same as second input
  Speed Limits (FWD only) : Saturate  UpperLimit=HIL_charge_nMax  LowerLimit=HIL_charge_nMin
  Sum : Sum  Inputs=|+-
  charge pump shaft speed (rpm) : Outport
  wires:
  Sum/1 -> PID Controller/1
  PID Controller/1 -> Speed Limits (FWD only)/1  "feedback cmd"
  pressure ref. (Pa)/1 -> Sum/1
  pressure meas. (Pa)/1 -> Sum/2
  Speed Limits (FWD only)/1 -> charge pump shaft speed (rpm)/1

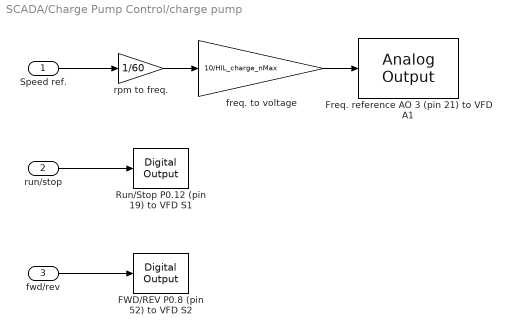
== system SCADA/Charge Pump Control/charge pump ==
  Speed ref. : Inport
  run/stop : Inport  Port=2
  fwd/rev : Inport  Port=3
  FWD/REV P0.8 (pin 52) to VFD S2 : sldrtlib/Digital Output  SampleTime=0.1  MaxMissedTicks=10  ShowMissedTicks=off  YieldWhenWaiting=off  DrvName=National_Instruments/PCIe-6343  DrvAddress=4294967295  DrvOptions=[0 4367 12288 3 3 3 3]  Channels=9  BitMode=1  InitialValue=0  FinalValue=0
      settings: AttributesFormatString=National Instruments\nPCIe-6343 [auto]  SourceProductBaseCode=WT
  "Freq. reference AO 3 (pin 21) to VFD A1 " : sldrtlib/Analog Output  SampleTime=0.1  MaxMissedTicks=inf  ShowMissedTicks=off  YieldWhenWaiting=off  DrvName=National_Instruments/PCIe-6343  DrvAddress=4294967295  DrvOptions=[0 4367 12288 3 3 3 3]  Channels=4  RangeMode=1  VoltRange=1  InitialValue=0  FinalValue=0
      settings: AttributesFormatString=National Instruments\nPCIe-6343 [auto]
  Run/Stop P0.12 (pin 19) to VFD S1 : sldrtlib/Digital Output  SampleTime=0.1  MaxMissedTicks=10  ShowMissedTicks=off  YieldWhenWaiting=off  DrvName=National_Instruments/PCIe-6343  DrvAddress=4294967295  DrvOptions=[0 4367 12288 3 3 3 3]  Channels=1  BitMode=1  InitialValue=[]  FinalValue=[]
      settings: AttributesFormatString=National Instruments\nPCIe-6343 [auto]  SourceProductBaseCode=WT
  freq. to voltage : Gain  Gain=10/HIL_charge_nMax
  rpm to freq. : Gain  Gain=1/60
  wires:
  Speed ref./1 -> rpm to freq./1
  rpm to freq./1 -> freq. to voltage/1
  freq. to voltage/1 -> "Freq. reference AO 3 (pin 21) to VFD A1 "/1
  run/stop/1 -> Run/Stop P0.12 (pin 19) to VFD S1/1
  fwd/rev/1 -> FWD/REV P0.8 (pin 52) to VFD S2/1

== system SCADA/ERU Control/ERU ==
  Speed ref. : Inport
  run/stop : Inport  Port=2
  fwd/rev : Inport  Port=3
  FWD/REV PFI 11/P2.3 (pin 46) to VFD S2 : sldrtlib/Digital Output  SampleTime=0.1  MaxMissedTicks=10  ShowMissedTicks=off  YieldWhenWaiting=off  DrvAddress=0  DrvOptions=0  Channels=1  BitMode=1  InitialValue=[]  FinalValue=[]
      settings: SourceProductBaseCode=WT
  "Freq. reference AO 0 (pin 22) to VFD A1 " : daqlib/Analog Output  DeviceMenu=(none)  Device=(none)  NChannelsSelected=1  NPorts=1 for all channels  SampleRate=0  ActualRate=0
      settings: SourceProductBaseCode=DA
  Run/Stop P0.3 (pin 47) to VFD S1 : sldrtlib/Digital Output  SampleTime=0.1  MaxMissedTicks=10  ShowMissedTicks=off  YieldWhenWaiting=off  DrvAddress=0  DrvOptions=0  Channels=1  BitMode=1  InitialValue=[]  FinalValue=[]
      settings: SourceProductBaseCode=WT
  freq. to voltage1 : Gain  Gain=10/HIL_ERU_nMax
  rpm to freq.1 : Gain  Gain=1/60
  wires:
  freq. to voltage1/1 -> "Freq. reference AO 0 (pin 22) to VFD A1 "/1
  run/stop/1 -> Run/Stop P0.3 (pin 47) to VFD S1/1
  fwd/rev/1 -> FWD/REV PFI 11/P2.3 (pin 46) to VFD S2/1
  rpm to freq.1/1 -> freq. to voltage1/1
  Speed ref./1 -> rpm to freq.1/1

== system SCADA/ERU Control/RO control ==
  recovery ref. : Inport
  recovery meas. : Inport  Port=2
  feed pressure (Pa) : Inport  Port=3
  PID Controller : slpidlib/PID Controller  Controller=PID  Form=Parallel  TimeDomain=Continuous-time  UseExternalTs=off  SampleTime=-1  IntegratorMethod=Forward Euler  FilterMethod=Forward Euler  ControllerParametersSource=internal  P=HIL_ERU_kp  I=HIL_ERU_ki  UseKiTs=off  D=HIL_ERU_kd  N=100  UseFilter=on  TunerSelectOption=Transfer Function Based (PID Tuner App)  InitialConditionSource=internal  InitialConditionForIntegrator=0  InitialConditionForFilter=0  DifferentiatorICPrevScaledInput=0  ExternalReset=none  TrackingMode=off  Kt=1  LimitOutput=off  SatLimitsSource=internal  UpperSaturationLimit=inf  LowerSaturationLimit=-inf  LinearizeAsGain=on  AntiWindupMode=none  Kb=1  POutMin=[]  POutMax=[]  IOutMin=[]  IOutMax=[]  DOutMin=[]  DOutMax=[]  NOutMin=[]  NOutMax=[]  SumOutMin=[]  SumOutMax=[]  SaturationOutMin=[]  SaturationOutMax=[]  PParamMin=[]  PParamMax=[]  IParamMin=[]  IParamMax=[]  DParamMin=[]  DParamMax=[]  NParamMin=[]  NParamMax=[]  KbParamMin=[]  KbParamMax=[]  KtParamMin=[]  KtParamMax=[]  KbOutMin=[]  KbOutMax=[]  KtOutMin=[]  KtOutMax=[]  IntegratorOutMin=[]  IntegratorOutMax=[]  FilterOutMin=[]  FilterOutMax=[]  SumI1OutMin=[]  SumI1OutMax=[]  SumI2OutMin=[]  SumI2OutMax=[]  SumI3OutMin=[]  SumI3OutMax=[]  SumI4OutMin=[]  SumI4OutMax=[]  SumDOutMin=[]  SumDOutMax=[]  DifferentiatorOutMin=[]  DifferentiatorOutMax=[]  FilterDiffOutCoefMin=[]  FilterDiffOutCoefMax=[]  ReciprocalOutMin=[]  ReciprocalOutMax=[]  SumDenOutMin=[]  SumDenOutMax=[]  SumNumOutMin=[]  SumNumOutMax=[]  DivideOutMin=[]  DivideOutMax=[]  UdiffTsProdOutMin=[]  UdiffTsProdOutMax=[]  NTsProdOutMin=[]  NTsProdOutMax=[]  UintegralTsProdOutMin=[]  UintegralTsProdOutMax=[]  UngainTsProdOutMin=[]  UngainTsProdOutMax=[]  IntegratorContinuousStateAttributes=''  IntegratorStateMustResolveToSignalObject=off  IntegratorRTWStateStorageClass=Auto  FilterContinuousStateAttributes=''  FilterStateMustResolveToSignalObject=off  FilterRTWStateStorageClass=Auto  ParallelPVariant=InternalParameters  IdealPVariant=Disabled  IVariant=InternalParameters  DVariant=InternalParameters  IntegratorVariant=Continuous  SatVariant=Disabled  AWVariant=Passthrough  PCopyVariant=Disabled  TRVariant=Disabled  FdbkBlocksVariant=Forward  IdealPFdbkVariant=Disabled  SatFdbkVariant=Disabled  DerivativeFilterVariant=ContFilter  NVariant=InternalParameters  NCopyVariant=Disabled  FilterICVariant=InternalICsFilter  IntegratorICVariant=InternalICs  ExternalResetVariant=Disabled  TRSumVariant=Passthrough  SumFdbkVariant=Disabled  SumVariant=Sum_PID  TsampFilterVariant=InternalTs  TsampNgainVariant=Passthrough  TsampIntegralVariant=Passthrough  ExternalSaturationOutDataTypeStr=Inherit: Same as second input  aMode=0
  Sum : Sum  Inputs=|+-
  Sum1 : Sum  Inputs=++|
  feed forward : MATLAB Function  TreatAsAtomicUnit=on
  ERU shaft speed (rpm) : Outport
  wires:
  Sum/1 -> PID Controller/1
  PID Controller/1 -> Sum1/2  "feedback cmd"
  recovery ref./1 -> feed forward/2(recoveryRef), Sum/1
  recovery meas./1 -> Sum/2
  feed pressure (Pa)/1 -> feed forward/1(pressure_feed)
  feed forward/1(shaftSpeedERU) -> Sum1/1
  Sum1/1 -> ERU shaft speed (rpm)/1

== system SCADA/Motor//Generator Control/RO feed pressure control ==
  feed pressure ref. (Pa) : Inport
  feed pressure meas. (Pa) : Inport  Port=2
  Feed forward : MATLAB Function  TreatAsAtomicUnit=on
  PID Controller : slpidlib/PID Controller  Controller=P  Form=Parallel  TimeDomain=Continuous-time  UseExternalTs=off  SampleTime=-1  IntegratorMethod=Forward Euler  FilterMethod=Forward Euler  ControllerParametersSource=internal  P=HIL_gen_kp  I=HIL_gen_ki  UseKiTs=off  D=HIL_gen_kd  N=100  UseFilter=on  TunerSelectOption=Transfer Function Based (PID Tuner App)  InitialConditionSource=internal  InitialConditionForIntegrator=0  InitialConditionForFilter=0  DifferentiatorICPrevScaledInput=0  ExternalReset=none  TrackingMode=off  Kt=1  LimitOutput=off  SatLimitsSource=internal  UpperSaturationLimit=inf  LowerSaturationLimit=-inf  LinearizeAsGain=on  AntiWindupMode=none  Kb=1  POutMin=[]  POutMax=[]  IOutMin=[]  IOutMax=[]  DOutMin=[]  DOutMax=[]  NOutMin=[]  NOutMax=[]  SumOutMin=[]  SumOutMax=[]  SaturationOutMin=[]  SaturationOutMax=[]  PParamMin=[]  PParamMax=[]  IParamMin=[]  IParamMax=[]  DParamMin=[]  DParamMax=[]  NParamMin=[]  NParamMax=[]  KbParamMin=[]  KbParamMax=[]  KtParamMin=[]  KtParamMax=[]  KbOutMin=[]  KbOutMax=[]  KtOutMin=[]  KtOutMax=[]  IntegratorOutMin=[]  IntegratorOutMax=[]  FilterOutMin=[]  FilterOutMax=[]  SumI1OutMin=[]  SumI1OutMax=[]  SumI2OutMin=[]  SumI2OutMax=[]  SumI3OutMin=[]  SumI3OutMax=[]  SumI4OutMin=[]  SumI4OutMax=[]  SumDOutMin=[]  SumDOutMax=[]  DifferentiatorOutMin=[]  DifferentiatorOutMax=[]  FilterDiffOutCoefMin=[]  FilterDiffOutCoefMax=[]  ReciprocalOutMin=[]  ReciprocalOutMax=[]  SumDenOutMin=[]  SumDenOutMax=[]  SumNumOutMin=[]  SumNumOutMax=[]  DivideOutMin=[]  DivideOutMax=[]  UdiffTsProdOutMin=[]  UdiffTsProdOutMax=[]  NTsProdOutMin=[]  NTsProdOutMax=[]  UintegralTsProdOutMin=[]  UintegralTsProdOutMax=[]  UngainTsProdOutMin=[]  UngainTsProdOutMax=[]  IntegratorContinuousStateAttributes=''  IntegratorStateMustResolveToSignalObject=off  IntegratorRTWStateStorageClass=Auto  FilterContinuousStateAttributes=''  FilterStateMustResolveToSignalObject=off  FilterRTWStateStorageClass=Auto  ParallelPVariant=InternalParameters  IdealPVariant=Disabled  IVariant=Disabled  DVariant=Disabled  IntegratorVariant=Disabled  SatVariant=Disabled  AWVariant=Disabled  PCopyVariant=Disabled  TRVariant=Disabled  FdbkBlocksVariant=Forward  IdealPFdbkVariant=Disabled  SatFdbkVariant=Disabled  DerivativeFilterVariant=Disabled  NVariant=Disabled  NCopyVariant=Disabled_SignalSpec  FilterICVariant=Disabled  IntegratorICVariant=Disabled  ExternalResetVariant=Disabled  TRSumVariant=Passthrough  SumFdbkVariant=Disabled  SumVariant=Passthrough_P  TsampFilterVariant=InternalTs  TsampNgainVariant=Passthrough  TsampIntegralVariant=Disabled_SignalSpec  ExternalSaturationOutDataTypeStr=Inherit: Same as second input  aMode=0
  Speed Limits (FWD only) : Saturate  UpperLimit=HIL_gen_nMax  LowerLimit=HIL_gen_nMin
  Sum : Sum  Inputs=|+-
  Sum1 : Sum  Inputs=++|
  gen shaft speed (rpm) : Outport
  wires:
  Sum/1 -> PID Controller/1
  PID Controller/1 -> Sum1/2  "feedback cmd"
  feed pressure ref. (Pa)/1 -> Feed forward/1(p), Sum/1
  feed pressure meas. (Pa)/1 -> Sum/2
  Speed Limits (FWD only)/1 -> gen shaft speed (rpm)/1
  Sum1/1 -> Speed Limits (FWD only)/1
  Feed forward/1(shaftSpeed_ff) -> Sum1/1

== system SCADA/Motor//Generator Control/generator ==
  Speed ref. : Inport
  run/stop : Inport  Port=2
  fwd/rev : Inport  Port=3
  FWD/REV P0.0 (pin 52) to VFD S2 : sldrtlib/Digital Output  SampleTime=0.1  MaxMissedTicks=10  ShowMissedTicks=off  YieldWhenWaiting=off  DrvAddress=0  DrvOptions=0  Channels=1  BitMode=1  InitialValue=[]  FinalValue=[]
      settings: SourceProductBaseCode=WT
  "Freq. reference AO 1 (pin 21) to VFD A1 " : daqlib/Analog Output  DeviceMenu=ni Dev1 (PCIe-6343)  Device=(none)  ObjConstructor=daq.createSession('ni')  NChannelsSelected=1  Channels=1$ao0$$Dev1$1$1$N/A$#1$ao1$$Dev1$1$1$N/A$#1$ao2$$Dev1$1$1$N/A$#1$ao3$$Dev1$1$1$N/A$#  NPorts=1 for all channels  SampleRate=0  ActualRate=0
      settings: SourceProductBaseCode=DA
  Run/Stop P0.4 (pin 19) to VFD S1 : sldrtlib/Digital Output  SampleTime=0.1  MaxMissedTicks=10  ShowMissedTicks=off  YieldWhenWaiting=off  DrvAddress=0  DrvOptions=0  Channels=1  BitMode=1  InitialValue=[]  FinalValue=[]
      settings: SourceProductBaseCode=WT
  freq. to voltage1 : Gain  Gain=10/HIL_gen_nMax
  rpm to freq.1 : Gain  Gain=1/60
  wires:
  Speed ref./1 -> rpm to freq.1/1
  run/stop/1 -> Run/Stop P0.4 (pin 19) to VFD S1/1
  fwd/rev/1 -> FWD/REV P0.0 (pin 52) to VFD S2/1
  rpm to freq.1/1 -> freq. to voltage1/1
  freq. to voltage1/1 -> "Freq. reference AO 1 (pin 21) to VFD A1 "/1

== system SCADA/Prescribed WEC-driven Pump Flow/Constant WEC-driven Pump Flow ==
  Gain : Gain  Gain=-1/HIL_WECpump_A_rod
  Gain1 : Gain  Gain=1/HIL_WECpump_A_cap
  Integrator : Integrator
  State Transition Table : State Transition Table  TreatAsAtomicUnit=on
  Switch : Switch  Criteria=u2 > Threshold
  pos. ref. : Outport
  vel. ref. : Outport  Port=2
  wires:
  Gain1/1 -> Switch/1
  Switch/1 -> vel. ref./1, Integrator/1
  Gain/1 -> Switch/3
  [NomFlow_WECpump] -> Gain1/1, Gain/1
  Integrator/1 -> State Transition Table/1(pos), pos. ref./1
  State Transition Table/1(direction) -> Switch/2

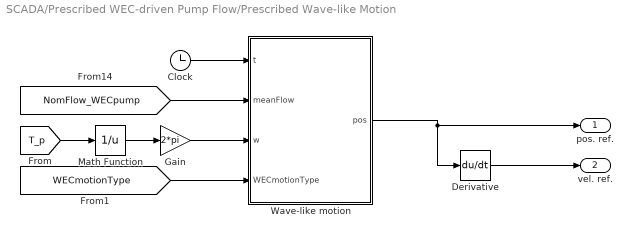
== system SCADA/Prescribed WEC-driven Pump Flow/Prescribed Wave-like Motion ==
  Clock : Clock
  Derivative : Derivative
  Gain : Gain  Gain=2*pi
  Math Function : Math  Operator=reciprocal  SaturateOnIntegerOverflow=on
  Wave-like motion : MATLAB Function  TreatAsAtomicUnit=on
  pos. ref. : Outport
  vel. ref. : Outport  Port=2
  wires:
  [NomFlow_WECpump] -> Wave-like motion/2(meanFlow)
  Wave-like motion/1(pos) -> Derivative/1, pos. ref./1
  Derivative/1 -> vel. ref./1
  Clock/1 -> Wave-like motion/1(t)
  [T_p] -> Math Function/1
  Math Function/1 -> Gain/1
  Gain/1 -> Wave-like motion/3(w)
  [WECmotionType] -> Wave-like motion/4(WECmotionType)

== stateflow chart SCADA/Prescribed WEC-driven Pump Flow/Constant WEC-driven Pump Flow/State Transition Table ==
  state forward
    entry:
    direction=1;
  state reverse
    entry:
    direction=0;
  (default) -> forward
  forward -> (junction 25) [order 2] : [pos<HIL_WECpump_positiveLimit]
  (junction 25) -> forward
  forward -> reverse [order 1] : [pos>=HIL_WECpump_positiveLimit]
  reverse -> forward [order 1] : [pos<=HIL_WECpump_negativeLimit]
  reverse -> (junction 29) [order 2] : [pos>HIL_WECpump_negativeLimit]
  (junction 29) -> reverse
  data: pos input; direction output; HIL_WECpump_negativeLimit parameter; HIL_WECpump_positiveLimit parameter

== matlab function SCADA/Prescribed WEC-driven Pump Flow/Prescribed Wave-like Motion/Wave-like motion ==
  data: t input; pos output; meanFlow input; w input; WECmotionType input; HIL_WECpump_A_cap parameter; HIL_WECpump_A_rod parameter
function pos = fcn(t,meanFlow,...
                w,WECmotionType,HIL_WECpump_A_cap, HIL_WECpump_A_rod)

% switch WECmotionType
%     case {0,1} % regular motion
        x_amp = meanFlow*pi/2/w/(HIL_WECpump_A_cap + HIL_WECpump_A_rod);
        
        pos = x_amp*sin(w*t);

%     case 1 % irregular motion
%         
%         pos = sum( x_amp.*sin(w.*t + psi));

% end

== matlab function SCADA/Motor//Generator Control/RO feed pressure control/Feed forward ==
  data: p input; shaftSpeed_ff output; HIL_charge_cn parameter
function shaftSpeed_ff = fcn(p,HIL_charge_cn)

shaftSpeed_ff = 60*swrt((p-1.013e5)/HIL_charge_cn);

== matlab function SCADA/Actuator Position//Velocity Control/Subsystem/MATLAB Function1 ==
  data: speed_rpm input; maxFlow_m3perSec output; numPumps input
function maxFlow_m3perSec = fcn(speed_rpm,numPumps)
displacement = 53.8; % [cc/rev]
maxFlow_m3perSec = numPumps*speed_rpm*60*displacement*1e-6;

== matlab function SCADA/Actuator Position//Velocity Control/Subsystem/MATLAB Function ==
  data: u input; dutyMag output; posCutIn input; negCutIn input; dutySign output
function [dutyMag,dutySign] = fcn(u,posCutIn,negCutIn)
duty = ((1-posCutIn)*u + posCutIn)*(u>0) + ...
    ((1-negCutIn)*u - negCutIn)*(u<0);
duty = max(-1,min(1,duty));
dutyMag = abs(duty);
dutySign = sign(duty);

== matlab function SCADA/Actuator Position//Velocity Control/Subsystem/FF flowrate ==
  data: vel_actuator input; flowrate output; HIL_act_A_cap parameter; HIL_act_A_rod parameter
function flowrate = fcn(vel_actuator,HIL_act_A_cap,HIL_act_A_rod)
flowrate = vel_actuator* ...
           (HIL_act_A_cap*(vel_actuator>=0) + ...
            HIL_act_A_rod*(vel_actuator<0));

== matlab function SCADA/ERU Control/RO control/feed forward ==
  data: pressure_feed input; shaftSpeedERU output; recoveryRef input
function shaftSpeedERU = fcn(pressure_feed,recoveryRef)
A_perm = 2.57e-12; % [m^3/(N-s)] permeability coeff.
S_perm = 33.6; % [m^3] membrane area
disp_ERUmotor = 9.31*1e-6; % [cc/rev -> m3/rev] motor displacement
effVol = 0.9;

q_perm = S_perm*A_perm*(pressure_feed - 2.7e6 - 101e3);
q_brineTarget = (1 - recoveryRef)*q_perm;

shaftSpeedERU = q_brineTarget/effVol/disp_ERUmotor*60;

== matlab function SCADA/WEC Simulation/Irregular Waves ==
  data: t input; waveElev output; T_e output; WEC_F_amp parameter; WEC_w parameter; WEC_dw parameter; WEC_phi_e parameter; wave_S_w parameter; wave_phi parameter
function [waveElev,T_e] = fcn(t, WEC_F_amp, WEC_w, WEC_dw, WEC_phi_e, wave_S_w, wave_phi)

T_e = sum( WEC_F_amp.*sqrt(2*wave_S_w.*WEC_dw) ...
            .*sin(WEC_w*t + wave_phi + WEC_phi_e ));

waveElev = sum( sqrt(2*wave_S_w(:).*WEC_dw) ...
                .*sin(WEC_w(:)*t + wave_phi(:)) );

== matlab function SCADA/WEC Simulation/Hydrostatic force ==
  data: pos input; T_h output; waveElev input; WEC_L_flap parameter; WEC_h parameter; WEC_T parameter; WEC_W parameter; rho parameter; g parameter; WEC_L_cm parameter; WEC_m parameter
function T_h = fcn(pos,waveElev,...
                    WEC_L_flap,WEC_h,WEC_T,WEC_W,rho, g, WEC_L_cm, WEC_m)
%% Determine buoyant torque from submerged volume

% Height of top edge of flap from hinge
h_top = WEC_L_flap*cos(pos);

% Length of submerged part of plate (by centerline) centroids 
% from thin plate assumption
L_sub = (h_top > WEC_h+waveElev)*(WEC_h+waveElev)/cos(pos) + ...
    (h_top <= WEC_h+waveElev)*WEC_L_flap; 

% Calculate the centroid of the buoyant force, position perpendicular to
% gravity
centroid_x = L_sub/2*sin(pos);

% calculate bouyant torque
T_buoy = WEC_T*L_sub*WEC_W*rho*g*centroid_x;

%% Determine torque due to off center weight
% Calculate position of the center of mass of the flap, perpendicular to
% gravity
cm_x = WEC_L_cm*sin(pos);

% calculate torque due to weight
T_weight = WEC_m*g*cm_x;

%% Determine total effective torque
T_h = T_buoy - T_weight;

== matlab function SCADA/WEC Simulation/Regular Waves ==
  data: t input; waveElev output; T_e output; WEC_F_amp parameter; WEC_w parameter; WEC_dw parameter; WEC_phi_e parameter; wave_S_w parameter; wave_phi parameter
function [waveElev,T_e] = fcn(t, WEC_F_amp, WEC_w, WEC_dw, WEC_phi_e, wave_S_w, wave_phi)

T_e = sum( WEC_F_amp.*sqrt(2*wave_S_w.*WEC_dw) ...
            .*sin(WEC_w*t + wave_phi + WEC_phi_e ));

waveElev = sum( sqrt(2*wave_S_w(:).*WEC_dw) ...
                .*sin(WEC_w(:)*t + wave_phi(:)) );
